simulink library "Springs_Axle3"  (R2026a)
settings: Solver=VariableStepAuto
undefined symbols (not defined in the file): Vehicle
libraries: Vehicle_Inputs x1, Springs_Axle3_Independent x1, Springs_Axle3_Interconnected x1, Springs_Axle3_Linear x1, Springs_Axle3_None x1
Description:
  | Component of Simscape Vehicle Templates Library
  | 
  | Copyright 2018-2026 The MathWorks, Inc.
settings Model: Creator=smiller  LastModifiedBy=smiller

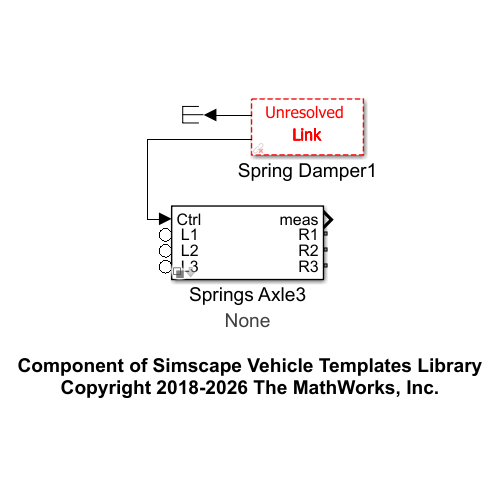
[thumbnail: Simulink's stored preview of the top-level diagram]
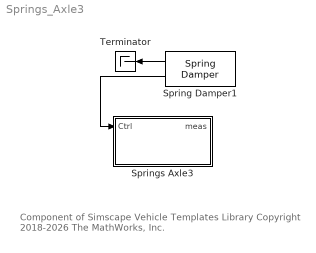
== system Springs_Axle3 ==
  note: Component of Simscape Vehicle Templates Library
      | Copyright 2018-2026 The MathWorks, Inc.
  Spring Damper1 : Vehicle_Inputs/Control Bus/Spring Damper  SystemSampleTime=-1  VariantActivationTime=update diagram  AllowFlexibleInterface=on  Latency=0  AutoFrameSizeCalculation=off
  Springs Axle3 : Subsystem  Variant=on  VariantControlMode=label  VariantControl=Variant1  LabelModeActiveChoice=None  mask(Variants for Springs){Spring=Vehicle.Chassis.Spring, VariantLabel=Vehicle.Chassis.Spring.class.Value}
      mask prompts: Spring "Spring Parameters"; VariantLabel "Variant Label"
      mask help: Select option and provide parameters for left and right springs on three axles. Option is chosen by string provided in Variant Label. The parameters for the selected option is contained in Springs data structure.
      mask init:
      | curblk = gcb;
      | 
      | % Set variant for this block 
      | set_param(curblk,'LabelModeActiveChoice',VariantLabel);
      settings: AttributesFormatString=%<ActiveVariant>
      mask Display:
      | if(strcmp(get_param(gcb,'LabelModeActiveChoice'),'None'))
      |     disp(' ');
      | else
      |     image('sm_car_vehicle_chassis_spring_IMAGE.png');
      | end
  Terminator : Terminator
  wires:
  Spring Damper1/1 -> Terminator/1
  Spring Damper1/2 -> Springs Axle3/1("Ctrl ")

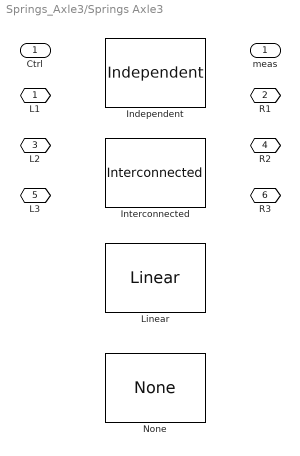
== system Springs_Axle3/Springs Axle3 ==
  "Ctrl " : Inport
  Independent : Springs_Axle3_Independent/Independent  VariantControl=Independent
  Interconnected : Springs_Axle3_Interconnected/Interconnected  VariantControl=Interconnected
  Linear : Springs_Axle3_Linear/Linear  SystemSampleTime=-1  VariantControl=Linear  VariantActivationTime=update diagram  EmptyChoice=off  PassThrough=off  PassThroughVariantControl=(default)  EmptyChoiceVariantControl=(default)  AllowFlexibleInterface=on  Latency=0  AutoFrameSizeCalculation=off
  None : Springs_Axle3_None/None  VariantControl=None
  " L1" : PMIOPort  Side=Left
  R1 : PMIOPort  Port=2  Side=Right
  " L2" : PMIOPort  Port=3  Side=Left
  R2 : PMIOPort  Port=4  Side=Right
  " L3" : PMIOPort  Port=5  Side=Left
  R3 : PMIOPort  Port=6  Side=Right
  " meas" : Outport  VectorParamsAs1DForOutWhenUnconnected=off
